simulink model "SIM_continuousFermenter"  (R2023b)
settings: Solver=VariableStepAuto  StartTime=0.0  StopTime=500  RelTol=1e-3
values from neighbouring files (symbols this model uses):
  Ts = 0.1    [MHE_compute.m]    (also in MHE_compute2.m; NMPC_conFer.m)
libraries: mpclib x1, simulink x1
settings Model: Creator=akeebismail  LastModifiedBy=akeebismail

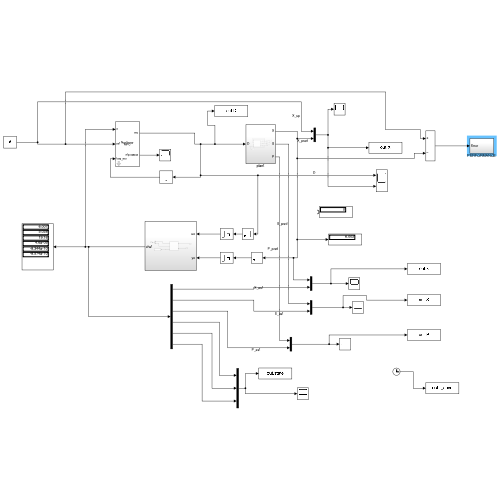
[thumbnail: Simulink's stored preview of the top-level diagram]
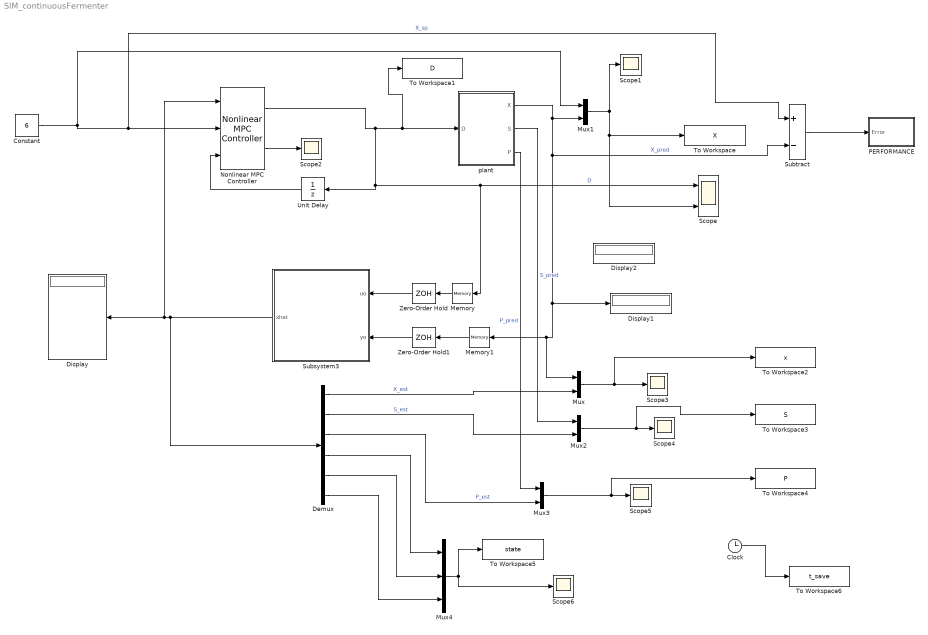
== system SIM_continuousFermenter ==
  Clock : Clock
  Constant : Constant  Value=6
  Demux : Demux  Outputs=6
  Display : Display
  Display1 : Display
  Display2 : Display
  Memory : Memory  InitialCondition=0.202
  Memory1 : Memory  InitialCondition=6
  Mux{,1..3} (4 alike) : Mux  Inputs=2
  Mux4 : Mux  Inputs=3
  Nonlinear MPC Controller : mpclib/Nonlinear MPC Controller  nlmpcobj=nlobj  UseObjectTs=on  UseMEX=off  md_enabled=off  mvtarget_enabled=off  param_enabled=off  cost_enabled=off  mvseq_enabled=off  stateseq_enabled=off  ovseq_enabled=off  slack_enabled=off  status_enabled=on  ov_min=off  ov_max=off  mv_min=off  mv_max=off  mvrate_min=off  mvrate_max=off  state_min=off  state_max=off  ov_weight=off  mv_weight=off  mvrate_weight=off  ecr_weight=off  nlp_initialize=off
  PERFORMANCE : Subsystem
  Scope : Scope  NumInputPorts=2
  Scope{1..6} (6 alike) : Scope
  Subsystem3 : Subsystem
  Subtract : Sum  Inputs=+-
  To Workspace : ToWorkspace  VariableName=X  SaveFormat=Timeseries  SampleTime=Ts
  To Workspace1 : ToWorkspace  VariableName=D  SaveFormat=Timeseries  SampleTime=Ts
  To Workspace2 : ToWorkspace  VariableName=x  SaveFormat=Timeseries  SampleTime=Ts
  To Workspace3 : ToWorkspace  VariableName=S  SaveFormat=Timeseries  SampleTime=Ts
  To Workspace4 : ToWorkspace  VariableName=P  SaveFormat=Timeseries  SampleTime=Ts
  To Workspace5 : ToWorkspace  VariableName=state  SaveFormat=Timeseries  SampleTime=Ts
  To Workspace6 : ToWorkspace  VariableName=t_save  SaveFormat=Timeseries  SampleTime=Ts
  Unit Delay : UnitDelay  InitialCondition=0.202  SampleTime=Ts  HasFrameUpgradeWarning=on
  Zero-Order Hold : ZeroOrderHold  SampleTime=Ts
  Zero-Order Hold1 : ZeroOrderHold  SampleTime=Ts
  plant : Subsystem
  wires:
  Nonlinear MPC Controller/1 -> Memory/1, Scope/1, Unit Delay/1, To Workspace1/1, plant/1(D)  "D"
  Constant/1 -> Subtract/1, Nonlinear MPC Controller/2, Mux1/1  "X_sp"
  Nonlinear MPC Controller/2 -> Scope2/1
  plant/1(X) -> Subtract/2, Memory1/1, Mux/1, Display1/1, Mux1/2  "X_pred"
  Unit Delay/1 -> Nonlinear MPC Controller/3
  Mux1/1 -> Scope/2, To Workspace/1, Scope1/1
  Subsystem3/1(xhat) -> Demux/1, Nonlinear MPC Controller/1, Display/1
  Zero-Order Hold/1 -> Subsystem3/1(uo)
  Mux/1 -> To Workspace2/1, Scope3/1
  Demux/1 -> Mux/2  "X_est"
  Zero-Order Hold1/1 -> Subsystem3/2(yo)
  Demux/3 -> Mux3/2  "P_est"
  Demux/2 -> Mux2/2  "S_est"
  plant/2(S) -> Mux2/1  "S_pred"
  plant/3(P) -> Mux3/1  "P_pred"
  Mux2/1 -> To Workspace3/1, Scope4/1
  Mux3/1 -> To Workspace4/1, Scope5/1
  Demux/4 -> Mux4/1
  Demux/5 -> Mux4/2
  Demux/6 -> Mux4/3
  Memory/1 -> Zero-Order Hold/1
  Memory1/1 -> Zero-Order Hold1/1
  Mux4/1 -> To Workspace5/1, Scope6/1
  Clock/1 -> To Workspace6/1
  Subtract/1 -> PERFORMANCE/1(Error)

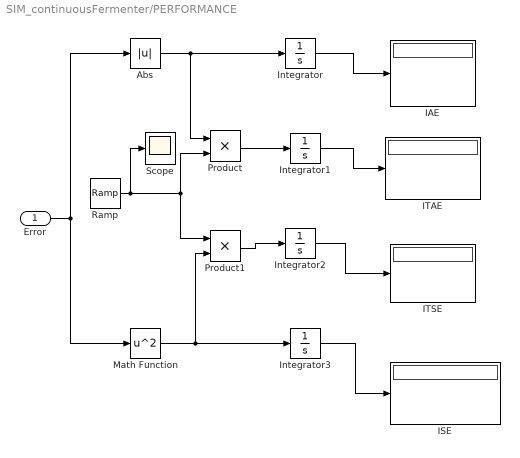
== system SIM_continuousFermenter/PERFORMANCE ==
  Error : Inport
  Abs : Abs  SaturateOnIntegerOverflow=off
  IAE : Display
  ISE : Display
  ITAE : Display
  ITSE : Display
  Integrator{,1..3} (4 alike) : Integrator
  Math Function : Math  Operator=square  SignedPower=on
  Product : Product  RndMeth=Zero
  Product1 : Product  RndMeth=Zero
  Ramp : simulink/Sources/Ramp  slope=1  start=0  InitialOutput=0
  Scope : Scope
  wires:
  Error/1 -> Math Function/1, Abs/1
  Abs/1 -> Integrator/1, Product/1
  Integrator/1 -> IAE/1
  Ramp/1 -> Product/2, Product1/1, Scope/1
  Math Function/1 -> Integrator3/1, Product1/2
  Product1/1 -> Integrator2/1
  Product/1 -> Integrator1/1
  Integrator3/1 -> ISE/1
  Integrator2/1 -> ITSE/1
  Integrator1/1 -> ITAE/1

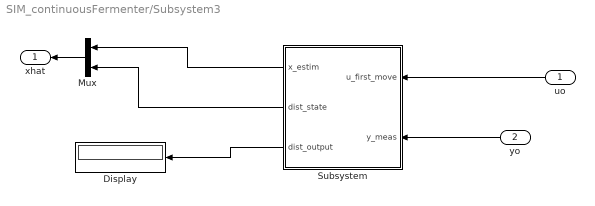
== system SIM_continuousFermenter/Subsystem3 ==
  uo : Inport
  yo : Inport  Port=2
  Display : Display
  Mux : Mux  Inputs=2
  Subsystem : Subsystem
  xhat : Outport
  wires:
  Subsystem/1(x_estim) -> Mux/1
  Subsystem/2(dist_state) -> Mux/2
  Subsystem/3(dist_output) -> Display/1
  uo/1 -> Subsystem/1(u_first_move)
  yo/1 -> Subsystem/2(y_meas)
  Mux/1 -> xhat/1

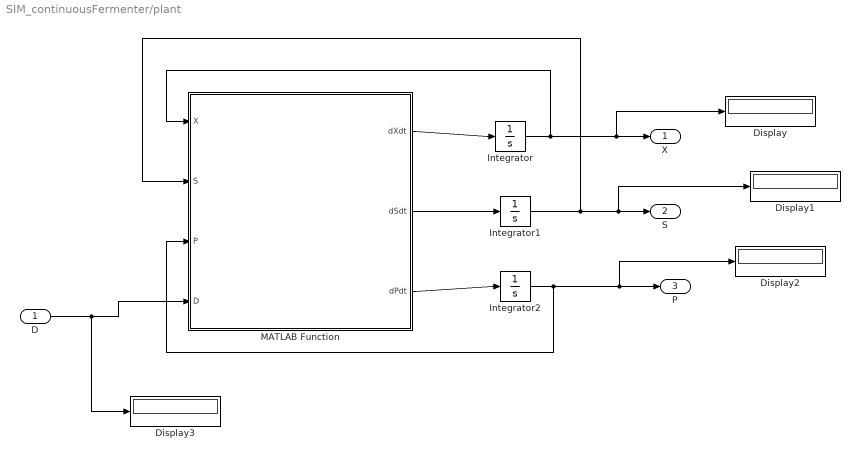
== system SIM_continuousFermenter/plant ==
  D : Inport
  Display{,1..3} (4 alike) : Display
  Integrator : Integrator  InitialCondition=5
  Integrator1 : Integrator  InitialCondition=5
  Integrator2 : Integrator  InitialCondition=19.14
  MATLAB Function : MATLAB Function  TreatAsAtomicUnit=on
  X : Outport
  S : Outport  Port=2
  P : Outport  Port=3
  wires:
  MATLAB Function/1(dXdt) -> Integrator/1
  MATLAB Function/3(dPdt) -> Integrator2/1
  MATLAB Function/2(dSdt) -> Integrator1/1
  D/1 -> Display3/1, MATLAB Function/4(D)
  Integrator/1 -> Display/1, X/1, MATLAB Function/1(X)
  Integrator2/1 -> Display2/1, P/1, MATLAB Function/3(P)
  Integrator1/1 -> Display1/1, S/1, MATLAB Function/2(S)

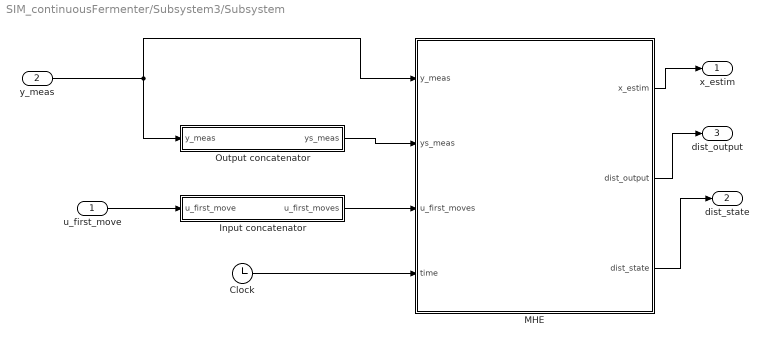
== system SIM_continuousFermenter/Subsystem3/Subsystem ==
  u_first_move : Inport  PortDimensions=[1,1]
  y_meas : Inport  Port=2  PortDimensions=[1,1]
  Clock : Clock
      settings: Decimation=20
  Input concatenator : Subsystem
  MHE : MATLAB Function  TreatAsAtomicUnit=on
  Output concatenator : Subsystem
  x_estim : Outport
  dist_state : Outport  Port=2
  dist_output : Outport  Port=3
  wires:
  Input concatenator/1(u_first_moves) -> MHE/3(u_first_moves)
  MHE/3(dist_state) -> dist_state/1
  MHE/2(dist_output) -> dist_output/1
  Clock/1 -> MHE/4(time)
  u_first_move/1 -> Input concatenator/1(u_first_move)
  MHE/1(x_estim) -> x_estim/1
  y_meas/1 -> MHE/1(y_meas), Output concatenator/1(y_meas)
  Output concatenator/1(ys_meas) -> MHE/2(ys_meas)

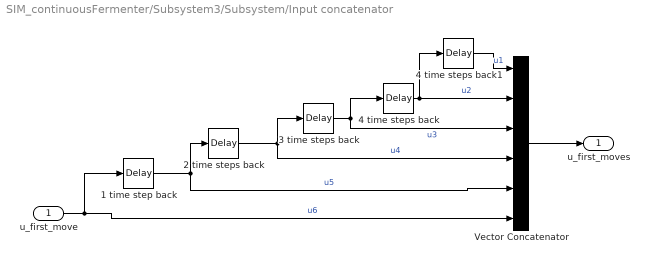
== system SIM_continuousFermenter/Subsystem3/Subsystem/Input concatenator ==
  u_first_move : Inport
  1 time step back : TransportDelay  DelayTime=0.1  InitialOutput=0.202
  2 time steps back : TransportDelay  DelayTime=0.1  InitialOutput=0.202
  3 time steps back : TransportDelay  DelayTime=0.1  InitialOutput=0.202
  4 time steps back : TransportDelay  DelayTime=0.1  InitialOutput=0.202
  4 time steps back1 : TransportDelay  DelayTime=0.1  InitialOutput=0.202
  Vector Concatenator : Concatenate  NumInputs=6  Mode=Multidimensional array
  u_first_moves : Outport  PortDimensions=[6,1]  VectorParamsAs1DForOutWhenUnconnected=off
  wires:
  Vector Concatenator/1 -> u_first_moves/1
  u_first_move/1 -> Vector Concatenator/6, 1 time step back/1  "u6"
  4 time steps back/1 -> Vector Concatenator/2, 4 time steps back1/1  "u2"
  3 time steps back/1 -> Vector Concatenator/3, 4 time steps back/1  "u3"
  2 time steps back/1 -> 3 time steps back/1, Vector Concatenator/4  "u4"
  1 time step back/1 -> 2 time steps back/1, Vector Concatenator/5  "u5"
  4 time steps back1/1 -> Vector Concatenator/1  "u1"

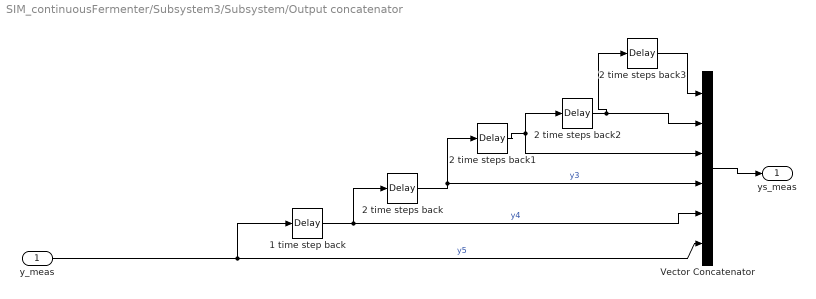
== system SIM_continuousFermenter/Subsystem3/Subsystem/Output concatenator ==
  y_meas : Inport
  1 time step back : TransportDelay  DelayTime=0.1  InitialOutput=6
  2 time steps back{,1..3} (4 alike) : TransportDelay  DelayTime=0.1  InitialOutput=6
  Vector Concatenator : Concatenate  NumInputs=6  Mode=Multidimensional array
  ys_meas : Outport  PortDimensions=[6,1]  VectorParamsAs1DForOutWhenUnconnected=off
  wires:
  2 time steps back2/1 -> 2 time steps back3/1, Vector Concatenator/2
  2 time steps back1/1 -> 2 time steps back2/1, Vector Concatenator/3
  Vector Concatenator/1 -> ys_meas/1
  2 time steps back/1 -> 2 time steps back1/1, Vector Concatenator/4  "y3"
  1 time step back/1 -> Vector Concatenator/5, 2 time steps back/1  "y4"
  y_meas/1 -> Vector Concatenator/6, 1 time step back/1  "y5"
  2 time steps back3/1 -> Vector Concatenator/1

== matlab function SIM_continuousFermenter/plant/MATLAB Function ==
  data: X input; dXdt output; S input; P input; D input; dSdt output; dPdt output
function [dXdt,dSdt,dPdt] = continuous_fermenter(X,S,P,D)

values = {22,1.2,50,20,0.4,2.2,0.2,0.48};

[Ki,Km,Pm,Sf,Yxs,alpha,beta,miu_m] = values{:};


miu = (miu_m * (1 - (P/Pm))) * S / (Km + S + (S^2 / Ki))  ;

dXdt = -D * X + miu * X     ;

dSdt = D * (Sf - S) - (1/Yxs) * miu * X   ;

dPdt = -D * P + (alpha * miu + beta) * X   ;

end

== matlab function SIM_continuousFermenter/Subsystem3/Subsystem/MHE ==
  data: y_meas input; ys_meas input; x_estim output; u_first_moves input; time input; dist_output output; dist_state output
function [x_estim,dist_output,dist_state] = MHE_4_tanks(y_meas,ys_meas,u_first_moves,time)

coder.extrinsic('MHE_compute2');

N_MHE=6  ;
% Ts=2 ;


if time < 5
    
    x_estim =  [6;5;19.14]  ;
   % x_estim = [17;17;17];
    %x_estim = [5.898;1.8];
    dist_output = 0;
    dist_state = [0;0;0];
else
    
    [x_estim,dist_state,dist_output] = MHE_compute2(ys_meas,u_first_moves,N_MHE,y_meas);
    %Note that our horizon must be constant here. It is chosen as 5.
end

end
